simulink model "test_filter"  (R2023a)
settings: Solver=ode4  StartTime=0.0  StopTime=1  FixedStep=0.001  RelTol=1e-3
values from neighbouring files (symbols this model uses):
  alpha = 0    [freq_sweep_continous.m]
undefined symbols (not defined in the file or in its folder): Discrete, Time
libraries: ctrlSharedLib x1
settings Model: Creator=dionl  LastModifiedBy=dionl

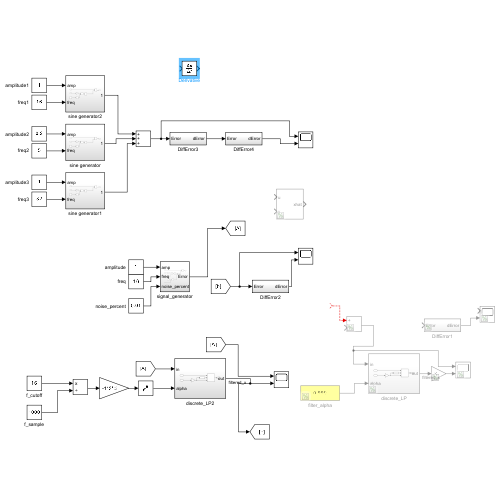
[thumbnail: Simulink's stored preview of the top-level diagram]
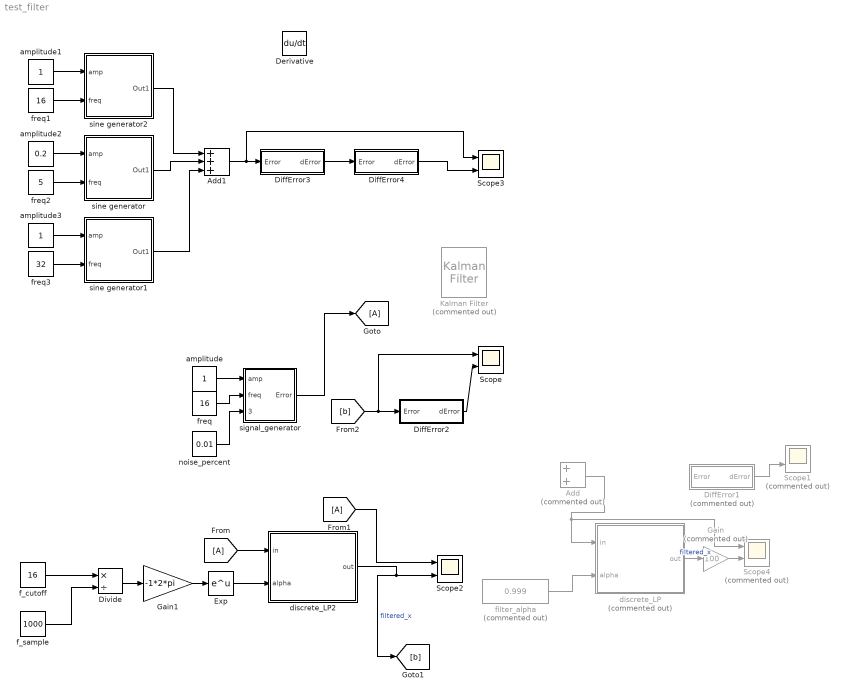
== system test_filter ==
  Add : Sum  Commented=on
  Add1 : Sum  Inputs=+++
  Derivative : Derivative
  DiffError1 : Subsystem  Commented=on
  DiffError2 : Subsystem
  DiffError3 : Subsystem
  DiffError4 : Subsystem
  Divide : Product  Inputs=*/
  Exp : Math
  From : From
  From1 : From
  Gain : Gain  Commented=on  Gain=100
  Gain1 : Gain  Gain=-1*2*pi
  Goto : Goto
  Kalman Filter : ctrlSharedLib/Kalman Filter  Commented=on  TimeDomain=Discrete-Time  UseCurrentEstimator=on  ModelSource=Individual A, B, C, D matrices  ModelSourceVariable=ss(0.95,1,1,0,1)  A=[0 1; 0 0]  B=[0; 0]  C=[1 0; 0 0]  D=[0; 0]  NumberOfStates=1  NumberOfInputs=1  NumberOfOutputs=1  InitialEstimateSource=Dialog  X0=0  P0=10  UseK=off  UseGH=off  NumberOfProcessNoiseInputs=1  G=1  TimeInvariantG=on  H=0  TimeInvariantH=on  Q=[1e-5 0; 0 1e-2]  TimeInvariantQ=on  R=diag([1e-4, 1e-2])  TimeInvariantR=on  N=0  TimeInvariantN=on  AddInputPort=on  AddEnablePort=off  OutputEstimatedY=off  OutputP=off  Ts=-1
  Scope : Scope  NumInputPorts=2
  Scope1 : Scope  Commented=on  NumInputPorts=2
  Scope2 : Scope  NumInputPorts=2
  Scope3 : Scope  NumInputPorts=2
  Scope4 : Scope  Commented=on  NumInputPorts=2
  amplitude : Constant
  amplitude1 : Constant
  amplitude2 : Constant  Value=0.2
  amplitude3 : Constant
  discrete_LP : Subsystem  Commented=on
  discrete_LP2 : Subsystem
  f_cutoff : Constant  Value=16
  f_sample : Constant  Value=1000
  filter_alpha : Constant  Commented=on  Value=0.999
  freq : Constant  Value=16
  freq1 : Constant  Value=16
  freq2 : Constant  Value=5
  freq3 : Constant  Value=32
  noise_percent : Constant  Value=0.01
  signal_generator : Subsystem
  sine generator : Subsystem
  sine generator1 : Subsystem
  sine generator2 : Subsystem
  wires:
  ? -> Add/1
  Gain/1 -> Scope4/2
  DiffError1/1(dError) -> Scope1/2
  filter_alpha/1 -> discrete_LP/2(alpha)
  discrete_LP/1(out) -> Gain/1  "filtered_x"
  Add/1 -> Scope4/1, discrete_LP/1(in)
  amplitude/1 -> signal_generator/1(amp)
  freq/1 -> signal_generator/2(freq)
  DiffError2/1(dError) -> Scope/2
  f_cutoff/1 -> Divide/1
  f_sample/1 -> Divide/2
  Divide/1 -> Gain1/1
  Gain1/1 -> Exp/1
  Exp/1 -> discrete_LP2/2(alpha)
  From/1 -> discrete_LP2/1(in)
  discrete_LP2/1(out) -> Scope2/2, [b]  "filtered_x"
  From1/1 -> Scope2/1
  noise_percent/1 -> signal_generator/3(noise_percent)
  freq1/1 -> sine generator2/2(freq)
  amplitude1/1 -> sine generator2/1(amp)
  amplitude2/1 -> sine generator/1(amp)
  freq2/1 -> sine generator/2(freq)
  amplitude3/1 -> sine generator1/1(amp)
  freq3/1 -> sine generator1/2(freq)
  sine generator2/1(Out1) -> Add1/1
  sine generator/1(Out1) -> Add1/2
  sine generator1/1(Out1) -> Add1/3
  signal_generator/1(Error) -> Goto/1
  [b] -> Scope/1, DiffError2/1(Error)
  Add1/1 -> Scope3/1, DiffError3/1(Error)
  DiffError3/1(dError) -> DiffError4/1(Error)
  DiffError4/1(dError) -> Scope3/2

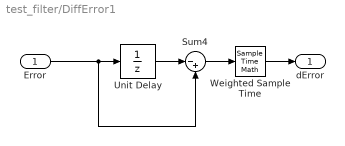
== system test_filter/DiffError1 ==
  Error : Inport
  Sum4 : Sum  Inputs=|-+
  Unit Delay : UnitDelay  SampleTime=-1  HasFrameUpgradeWarning=on
  Weighted Sample Time : SampleTimeMath  TsampMathOp=/
  dError : Outport
  wires:
  Error/1 -> Sum4/2, Unit Delay/1
  Weighted Sample Time/1 -> dError/1
  Sum4/1 -> Weighted Sample Time/1
  Unit Delay/1 -> Sum4/1

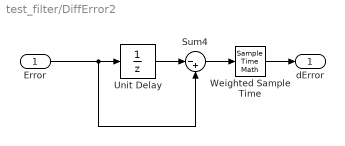
== system test_filter/DiffError2 ==
  Error : Inport
  Sum4 : Sum  Inputs=|-+
  Unit Delay : UnitDelay  SampleTime=-1  HasFrameUpgradeWarning=on
  Weighted Sample Time : SampleTimeMath  TsampMathOp=/
  dError : Outport
  wires:
  Unit Delay/1 -> Sum4/1
  Sum4/1 -> Weighted Sample Time/1
  Weighted Sample Time/1 -> dError/1
  Error/1 -> Unit Delay/1, Sum4/2

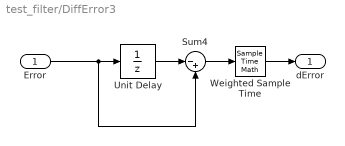
== system test_filter/DiffError3 ==
  Error : Inport
  Sum4 : Sum  Inputs=|-+
  Unit Delay : UnitDelay  SampleTime=-1  HasFrameUpgradeWarning=on
  Weighted Sample Time : SampleTimeMath  TsampMathOp=/
  dError : Outport
  wires:
  Error/1 -> Sum4/2, Unit Delay/1
  Weighted Sample Time/1 -> dError/1
  Sum4/1 -> Weighted Sample Time/1
  Unit Delay/1 -> Sum4/1

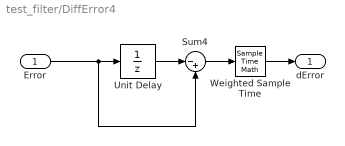
== system test_filter/DiffError4 ==
  Error : Inport
  Sum4 : Sum  Inputs=|-+
  Unit Delay : UnitDelay  SampleTime=-1  HasFrameUpgradeWarning=on
  Weighted Sample Time : SampleTimeMath  TsampMathOp=/
  dError : Outport
  wires:
  Unit Delay/1 -> Sum4/1
  Sum4/1 -> Weighted Sample Time/1
  Weighted Sample Time/1 -> dError/1
  Error/1 -> Unit Delay/1, Sum4/2

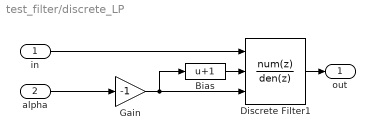
== system test_filter/discrete_LP ==
  in : Inport
  alpha : Inport  Port=2
  Bias : Bias  Bias=1  SaturateOnIntegerOverflow=off
  Discrete Filter1 : DiscreteFilter  NumeratorSource=Input port  Numerator=[1-alpha]  DenominatorSource=Input port  Denominator=[1, alpha]  a0EqualsOne=on
      settings: InputPortMap=u0,p1,p3
  Gain : Gain  Gain=-1
  out : Outport
  wires:
  Gain/1 -> Bias/1, Discrete Filter1/3
  Bias/1 -> Discrete Filter1/2
  in/1 -> Discrete Filter1/1
  Discrete Filter1/1 -> out/1
  alpha/1 -> Gain/1

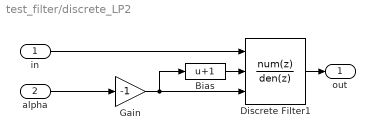
== system test_filter/discrete_LP2 ==
  in : Inport
  alpha : Inport  Port=2
  Bias : Bias  Bias=1  SaturateOnIntegerOverflow=off
  Discrete Filter1 : DiscreteFilter  NumeratorSource=Input port  Numerator=[1-alpha]  DenominatorSource=Input port  Denominator=[1, alpha]  a0EqualsOne=on
      settings: InputPortMap=u0,p1,p3
  Gain : Gain  Gain=-1
  out : Outport
  wires:
  alpha/1 -> Gain/1
  Discrete Filter1/1 -> out/1
  in/1 -> Discrete Filter1/1
  Bias/1 -> Discrete Filter1/2
  Gain/1 -> Discrete Filter1/3, Bias/1

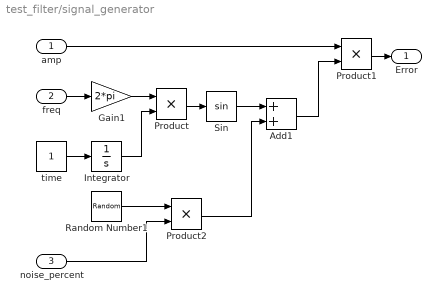
== system test_filter/signal_generator ==
  amp : Inport
  freq : Inport  Port=2
  noise_percent : Inport  Port=3
  Add1 : Sum
  Gain1 : Gain  Gain=2*pi
  Integrator : Integrator
  Product : Product
  Product1 : Product
  Product2 : Product
  Random Number1 : RandomNumber  SampleTime=0.001
  Sin : Trigonometry
  time : Constant
  Error : Outport
  wires:
  Gain1/1 -> Product/1
  amp/1 -> Product1/1
  Sin/1 -> Add1/1
  Product2/1 -> Add1/2
  Add1/1 -> Product1/2
  Integrator/1 -> Product/2
  Product/1 -> Sin/1
  Random Number1/1 -> Product2/1
  time/1 -> Integrator/1
  freq/1 -> Gain1/1
  Product1/1 -> Error/1
  noise_percent/1 -> Product2/2

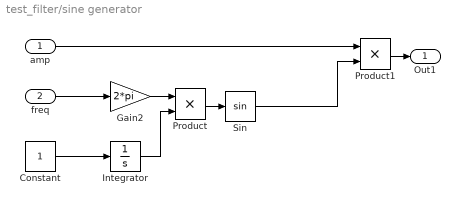
== system test_filter/sine generator ==
  amp : Inport
  freq : Inport  Port=2
  Constant : Constant
  Gain2 : Gain  Gain=2*pi
  Integrator : Integrator
  Product : Product
  Product1 : Product
  Sin : Trigonometry
  Out1 : Outport
  wires:
  Product1/1 -> Out1/1
  Product/1 -> Sin/1
  Constant/1 -> Integrator/1
  freq/1 -> Gain2/1
  Gain2/1 -> Product/1
  Integrator/1 -> Product/2
  Sin/1 -> Product1/2
  amp/1 -> Product1/1

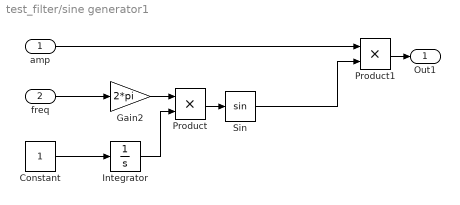
== system test_filter/sine generator1 ==
  amp : Inport
  freq : Inport  Port=2
  Constant : Constant
  Gain2 : Gain  Gain=2*pi
  Integrator : Integrator
  Product : Product
  Product1 : Product
  Sin : Trigonometry
  Out1 : Outport
  wires:
  amp/1 -> Product1/1
  Sin/1 -> Product1/2
  Integrator/1 -> Product/2
  Gain2/1 -> Product/1
  freq/1 -> Gain2/1
  Constant/1 -> Integrator/1
  Product/1 -> Sin/1
  Product1/1 -> Out1/1

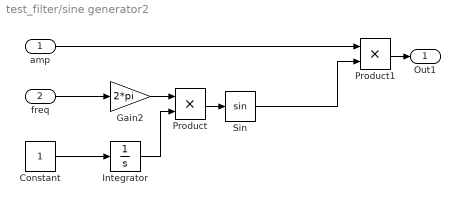
== system test_filter/sine generator2 ==
  amp : Inport
  freq : Inport  Port=2
  Constant : Constant
  Gain2 : Gain  Gain=2*pi
  Integrator : Integrator
  Product : Product
  Product1 : Product
  Sin : Trigonometry
  Out1 : Outport
  wires:
  Product1/1 -> Out1/1
  Product/1 -> Sin/1
  Constant/1 -> Integrator/1
  freq/1 -> Gain2/1
  Gain2/1 -> Product/1
  Integrator/1 -> Product/2
  Sin/1 -> Product1/2
  amp/1 -> Product1/1
